simulink model "TST_AccPed_DrvDemLead"  (R2016b)
settings: Solver=FixedStepDiscrete  StartTime=0.0  StopTime=simTime  FixedStep=sampleTime  RelTol=1e-3
values from neighbouring files (symbols this model uses):
  testCase = 1    [initTST_AccPed_DrvDemLead_001.m]    (also in initTST_AccPed_DrvDemLead_002.m = 2; initTST_AccPed_DrvDemLead_003.m = 3; initTST_AccPed_DrvDemLead_004.m = 4)
libraries: simulink x17, UnitTest_Lib x12
settings Model: Creator=zhengjinyan  LastModifiedBy=zhengjinyan
settings DebuggingCC: SignalRangeChecking=error

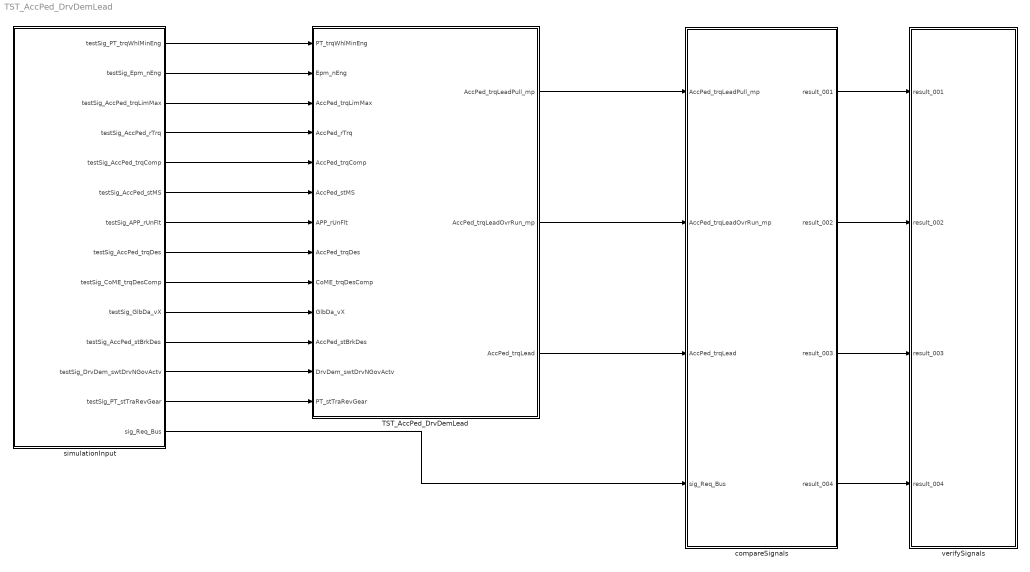
== system TST_AccPed_DrvDemLead ==
  TST_AccPed_DrvDemLead : Subsystem
  compareSignals : Subsystem
  simulationInput : Subsystem
  verifySignals : Subsystem
  wires:
  simulationInput/1(testSig_PT_trqWhlMinEng) -> TST_AccPed_DrvDemLead/1(PT_trqWhlMinEng)
  simulationInput/2(testSig_Epm_nEng) -> TST_AccPed_DrvDemLead/2(Epm_nEng)
  simulationInput/3(testSig_AccPed_trqLimMax) -> TST_AccPed_DrvDemLead/3(AccPed_trqLimMax)
  simulationInput/4(testSig_AccPed_rTrq) -> TST_AccPed_DrvDemLead/4(AccPed_rTrq)
  simulationInput/5(testSig_AccPed_trqComp) -> TST_AccPed_DrvDemLead/5(AccPed_trqComp)
  simulationInput/6(testSig_AccPed_stMS) -> TST_AccPed_DrvDemLead/6(AccPed_stMS)
  simulationInput/7(testSig_APP_rUnFlt) -> TST_AccPed_DrvDemLead/7(APP_rUnFlt)
  simulationInput/8(testSig_AccPed_trqDes) -> TST_AccPed_DrvDemLead/8(AccPed_trqDes)
  simulationInput/9(testSig_CoME_trqDesComp) -> TST_AccPed_DrvDemLead/9(CoME_trqDesComp)
  simulationInput/10(testSig_GlbDa_vX) -> TST_AccPed_DrvDemLead/10(GlbDa_vX)
  simulationInput/11(testSig_AccPed_stBrkDes) -> TST_AccPed_DrvDemLead/11(AccPed_stBrkDes)
  simulationInput/12(testSig_DrvDem_swtDrvNGovActv) -> TST_AccPed_DrvDemLead/12(DrvDem_swtDrvNGovActv)
  simulationInput/13(testSig_PT_stTraRevGear) -> TST_AccPed_DrvDemLead/13(PT_stTraRevGear)
  TST_AccPed_DrvDemLead/1(AccPed_trqLeadPull_mp) -> compareSignals/1(AccPed_trqLeadPull_mp)
  TST_AccPed_DrvDemLead/2(AccPed_trqLeadOvrRun_mp) -> compareSignals/2(AccPed_trqLeadOvrRun_mp)
  TST_AccPed_DrvDemLead/3(AccPed_trqLead) -> compareSignals/3(AccPed_trqLead)
  simulationInput/14(sig_Req_Bus) -> compareSignals/4(sig_Req_Bus)
  compareSignals/1(result_001) -> verifySignals/1(result_001)
  compareSignals/2(result_002) -> verifySignals/2(result_002)
  compareSignals/3(result_003) -> verifySignals/3(result_003)
  compareSignals/4(result_004) -> verifySignals/4(result_004)

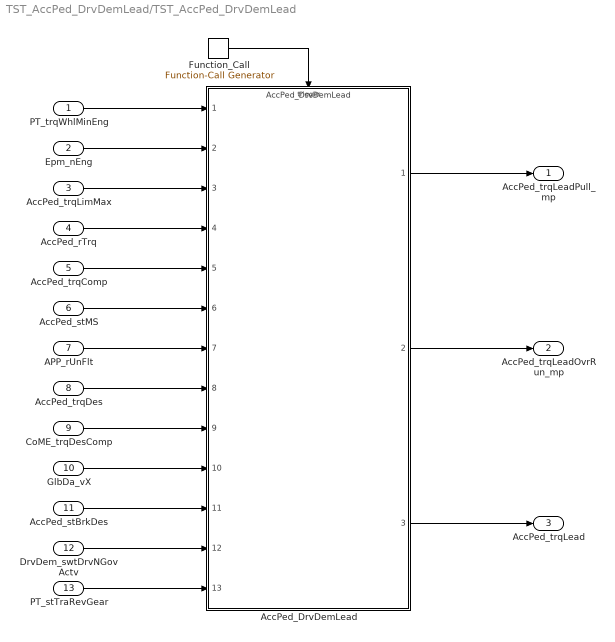
== system TST_AccPed_DrvDemLead/TST_AccPed_DrvDemLead ==
  PT_trqWhlMinEng : Inport
  Epm_nEng : Inport  Port=2
  AccPed_trqLimMax : Inport  Port=3
  AccPed_rTrq : Inport  Port=4
  AccPed_trqComp : Inport  Port=5
  AccPed_stMS : Inport  Port=6
  APP_rUnFlt : Inport  Port=7
  AccPed_trqDes : Inport  Port=8
  CoME_trqDesComp : Inport  Port=9
  GlbDa_vX : Inport  Port=10
  AccPed_stBrkDes : Inport  Port=11
  DrvDem_swtDrvNGovActv : Inport  Port=12
  PT_stTraRevGear : Inport  Port=13
  AccPed_DrvDemLead : ModelReference  ModelNameDialog=AccPed_DrvDemLead  SimulationMode=Normal  ModelReferenceVersion=1.27  TriggerPortName=function  TriggerPortTriggerType=function-call  TriggerPortStatesWhenEnabling=held
  Function_Call : simulink/Ports & Subsystems/Function-Call Generator  sample_time=sampleTime  numberOfIterations=1
  AccPed_trqLeadPull_mp : Outport
  AccPed_trqLeadOvrRun_mp : Outport  Port=2
  AccPed_trqLead : Outport  Port=3
  wires:
  Function_Call/1 -> AccPed_DrvDemLead/Trigger
  PT_trqWhlMinEng/1 -> AccPed_DrvDemLead/1
  Epm_nEng/1 -> AccPed_DrvDemLead/2
  AccPed_trqLimMax/1 -> AccPed_DrvDemLead/3
  AccPed_rTrq/1 -> AccPed_DrvDemLead/4
  AccPed_trqComp/1 -> AccPed_DrvDemLead/5
  AccPed_stMS/1 -> AccPed_DrvDemLead/6
  APP_rUnFlt/1 -> AccPed_DrvDemLead/7
  AccPed_trqDes/1 -> AccPed_DrvDemLead/8
  CoME_trqDesComp/1 -> AccPed_DrvDemLead/9
  GlbDa_vX/1 -> AccPed_DrvDemLead/10
  AccPed_stBrkDes/1 -> AccPed_DrvDemLead/11
  DrvDem_swtDrvNGovActv/1 -> AccPed_DrvDemLead/12
  PT_stTraRevGear/1 -> AccPed_DrvDemLead/13
  AccPed_DrvDemLead/1 -> AccPed_trqLeadPull_mp/1
  AccPed_DrvDemLead/2 -> AccPed_trqLeadOvrRun_mp/1
  AccPed_DrvDemLead/3 -> AccPed_trqLead/1

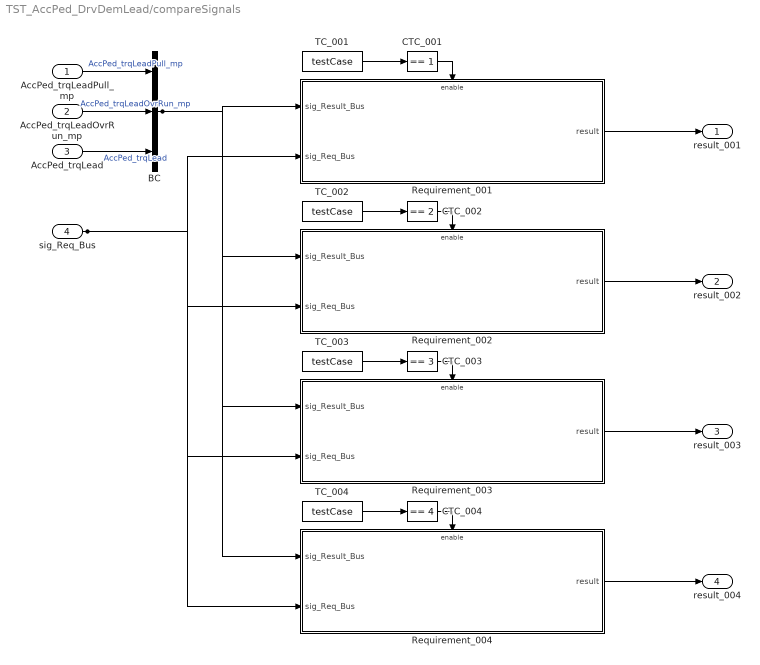
== system TST_AccPed_DrvDemLead/compareSignals ==
  AccPed_trqLeadPull_mp : Inport
  AccPed_trqLeadOvrRun_mp : Inport  Port=2
  AccPed_trqLead : Inport  Port=3
  sig_Req_Bus : Inport  Port=4
  BC : BusCreator  Inputs=3
  CTC_001 : simulink/Logic and Bit Operations/Compare To Constant  relop===  const=1  OutDataTypeStr=boolean
  CTC_002 : simulink/Logic and Bit Operations/Compare To Constant  relop===  const=2  OutDataTypeStr=boolean
  CTC_003 : simulink/Logic and Bit Operations/Compare To Constant  relop===  const=3  OutDataTypeStr=boolean
  CTC_004 : simulink/Logic and Bit Operations/Compare To Constant  relop===  const=4  OutDataTypeStr=boolean
  Requirement_001 : Subsystem
  Requirement_002 : Subsystem
  Requirement_003 : Subsystem
  Requirement_004 : Subsystem
  TC_001 : Constant  Value=testCase
  TC_002 : Constant  Value=testCase
  TC_003 : Constant  Value=testCase
  TC_004 : Constant  Value=testCase
  result_001 : Outport
  result_002 : Outport  Port=2
  result_003 : Outport  Port=3
  result_004 : Outport  Port=4
  wires:
  AccPed_trqLeadPull_mp/1 -> BC/1  "AccPed_trqLeadPull_mp"
  AccPed_trqLeadOvrRun_mp/1 -> BC/2  "AccPed_trqLeadOvrRun_mp"
  AccPed_trqLead/1 -> BC/3  "AccPed_trqLead"
  TC_001/1 -> CTC_001/1
  CTC_001/1 -> Requirement_001/Enable
  sig_Req_Bus/1 -> Requirement_001/2(sig_Req_Bus), Requirement_002/2(sig_Req_Bus), Requirement_003/2(sig_Req_Bus), Requirement_004/2(sig_Req_Bus)
  BC/1 -> Requirement_001/1(sig_Result_Bus), Requirement_002/1(sig_Result_Bus), Requirement_003/1(sig_Result_Bus), Requirement_004/1(sig_Result_Bus)
  Requirement_001/1(result) -> result_001/1
  TC_002/1 -> CTC_002/1
  CTC_002/1 -> Requirement_002/Enable
  Requirement_002/1(result) -> result_002/1
  TC_003/1 -> CTC_003/1
  CTC_003/1 -> Requirement_003/Enable
  Requirement_003/1(result) -> result_003/1
  TC_004/1 -> CTC_004/1
  CTC_004/1 -> Requirement_004/Enable
  Requirement_004/1(result) -> result_004/1

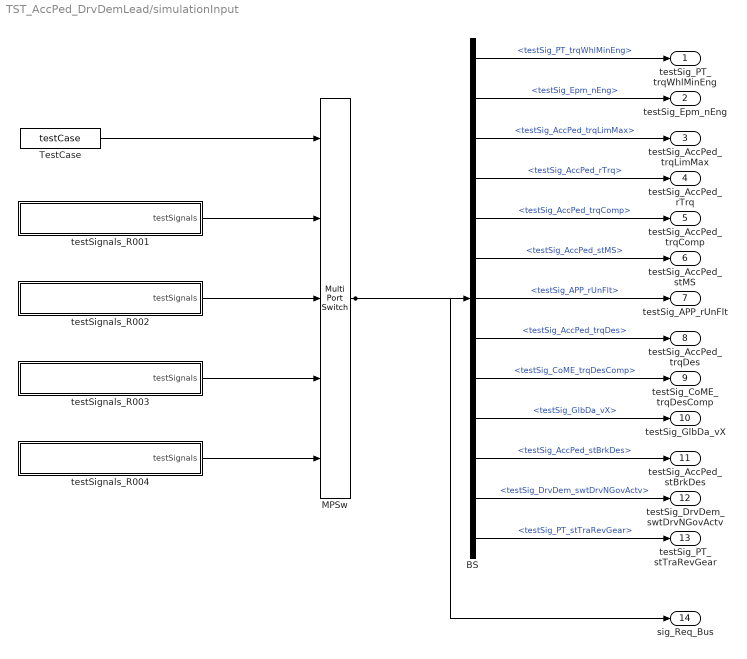
== system TST_AccPed_DrvDemLead/simulationInput ==
  BS : BusSelector  OutputSignals=testSig_PT_trqWhlMinEng,testSig_Epm_nEng,testSig_AccPed_trqLimMax,testSig_AccPed_rTrq,testSig_AccPed_trqComp,testSig_AccPed_stMS,testSig_APP_rUnFlt,testSig_AccPed_trqDes,testSig_CoME_trqDesComp,testSig_GlbDa_vX,testSig_AccPed_stBrkDes,testSig_DrvDem_swtDrvNGovActv,testSig_PT_stTraRevGear
  MPSw : MultiPortSwitch  Inputs=4  SaturateOnIntegerOverflow=on  InputSameDT=on
  TestCase : Constant  Value=testCase
  testSignals_R001 : Subsystem
  testSignals_R002 : Subsystem
  testSignals_R003 : Subsystem
  testSignals_R004 : Subsystem
  testSig_PT_trqWhlMinEng : Outport
  testSig_Epm_nEng : Outport  Port=2
  testSig_AccPed_trqLimMax : Outport  Port=3
  testSig_AccPed_rTrq : Outport  Port=4
  testSig_AccPed_trqComp : Outport  Port=5
  testSig_AccPed_stMS : Outport  Port=6
  testSig_APP_rUnFlt : Outport  Port=7
  testSig_AccPed_trqDes : Outport  Port=8
  testSig_CoME_trqDesComp : Outport  Port=9
  testSig_GlbDa_vX : Outport  Port=10
  testSig_AccPed_stBrkDes : Outport  Port=11
  testSig_DrvDem_swtDrvNGovActv : Outport  Port=12
  testSig_PT_stTraRevGear : Outport  Port=13
  sig_Req_Bus : Outport  Port=14
  wires:
  BS/1 -> testSig_PT_trqWhlMinEng/1  "<testSig_PT_trqWhlMinEng>"
  BS/2 -> testSig_Epm_nEng/1  "<testSig_Epm_nEng>"
  BS/3 -> testSig_AccPed_trqLimMax/1  "<testSig_AccPed_trqLimMax>"
  BS/4 -> testSig_AccPed_rTrq/1  "<testSig_AccPed_rTrq>"
  BS/5 -> testSig_AccPed_trqComp/1  "<testSig_AccPed_trqComp>"
  BS/6 -> testSig_AccPed_stMS/1  "<testSig_AccPed_stMS>"
  BS/7 -> testSig_APP_rUnFlt/1  "<testSig_APP_rUnFlt>"
  BS/8 -> testSig_AccPed_trqDes/1  "<testSig_AccPed_trqDes>"
  BS/9 -> testSig_CoME_trqDesComp/1  "<testSig_CoME_trqDesComp>"
  BS/10 -> testSig_GlbDa_vX/1  "<testSig_GlbDa_vX>"
  BS/11 -> testSig_AccPed_stBrkDes/1  "<testSig_AccPed_stBrkDes>"
  BS/12 -> testSig_DrvDem_swtDrvNGovActv/1  "<testSig_DrvDem_swtDrvNGovActv>"
  BS/13 -> testSig_PT_stTraRevGear/1  "<testSig_PT_stTraRevGear>"
  MPSw/1 -> BS/1, sig_Req_Bus/1
  TestCase/1 -> MPSw/1
  testSignals_R001/1(testSignals) -> MPSw/2
  testSignals_R002/1(testSignals) -> MPSw/3
  testSignals_R003/1(testSignals) -> MPSw/4
  testSignals_R004/1(testSignals) -> MPSw/5

== system TST_AccPed_DrvDemLead/verifySignals ==
  result_001 : Inport
  result_002 : Inport  Port=2
  result_003 : Inport  Port=3
  result_004 : Inport  Port=4
  Assertion_001 : Assertion  Enabled=off
  Assertion_002 : Assertion  Enabled=off
  Assertion_003 : Assertion  Enabled=off
  Assertion_004 : Assertion  Enabled=off
  wires:
  result_001/1 -> Assertion_001/1
  result_002/1 -> Assertion_002/1
  result_003/1 -> Assertion_003/1
  result_004/1 -> Assertion_004/1

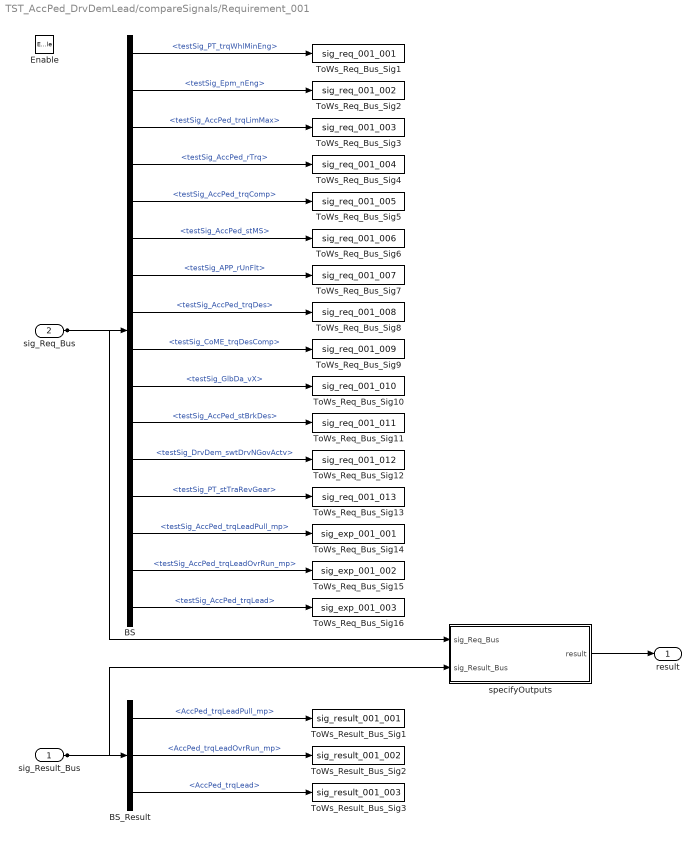
== system TST_AccPed_DrvDemLead/compareSignals/Requirement_001 ==
  sig_Result_Bus : Inport
  sig_Req_Bus : Inport  Port=2
  Enable : EnablePort
  BS : BusSelector  OutputSignals=testSig_PT_trqWhlMinEng,testSig_Epm_nEng,testSig_AccPed_trqLimMax,testSig_AccPed_rTrq,testSig_AccPed_trqComp,testSig_AccPed_stMS,testSig_APP_rUnFlt,testSig_AccPed_trqDes,testSig_CoME_trqDesComp,testSig_GlbDa_vX,testSig_AccPed_stBrkDes,testSig_DrvDem_swtDrvNGovActv,testSig_PT_stTraRevGear,testSig_AccPed_trqLeadPull_mp,testSig_AccPed_trqLeadOvrRun_mp,testSig_AccPed_trqLead
  BS_Result : BusSelector  OutputSignals=AccPed_trqLeadPull_mp,AccPed_trqLeadOvrRun_mp,AccPed_trqLead
  ToWs_Req_Bus_Sig1 : ToWorkspace  VariableName=sig_req_001_001  SaveFormat=Structure With Time
  ToWs_Req_Bus_Sig10 : ToWorkspace  VariableName=sig_req_001_010  SaveFormat=Structure With Time
  ToWs_Req_Bus_Sig11 : ToWorkspace  VariableName=sig_req_001_011  SaveFormat=Structure With Time
  ToWs_Req_Bus_Sig12 : ToWorkspace  VariableName=sig_req_001_012  SaveFormat=Structure With Time
  ToWs_Req_Bus_Sig13 : ToWorkspace  VariableName=sig_req_001_013  SaveFormat=Structure With Time
  ToWs_Req_Bus_Sig14 : ToWorkspace  VariableName=sig_exp_001_001  SaveFormat=Structure With Time
  ToWs_Req_Bus_Sig15 : ToWorkspace  VariableName=sig_exp_001_002  SaveFormat=Structure With Time
  ToWs_Req_Bus_Sig16 : ToWorkspace  VariableName=sig_exp_001_003  SaveFormat=Structure With Time
  ToWs_Req_Bus_Sig2 : ToWorkspace  VariableName=sig_req_001_002  SaveFormat=Structure With Time
  ToWs_Req_Bus_Sig3 : ToWorkspace  VariableName=sig_req_001_003  SaveFormat=Structure With Time
  ToWs_Req_Bus_Sig4 : ToWorkspace  VariableName=sig_req_001_004  SaveFormat=Structure With Time
  ToWs_Req_Bus_Sig5 : ToWorkspace  VariableName=sig_req_001_005  SaveFormat=Structure With Time
  ToWs_Req_Bus_Sig6 : ToWorkspace  VariableName=sig_req_001_006  SaveFormat=Structure With Time
  ToWs_Req_Bus_Sig7 : ToWorkspace  VariableName=sig_req_001_007  SaveFormat=Structure With Time
  ToWs_Req_Bus_Sig8 : ToWorkspace  VariableName=sig_req_001_008  SaveFormat=Structure With Time
  ToWs_Req_Bus_Sig9 : ToWorkspace  VariableName=sig_req_001_009  SaveFormat=Structure With Time
  ToWs_Result_Bus_Sig1 : ToWorkspace  VariableName=sig_result_001_001  SaveFormat=Structure With Time
  ToWs_Result_Bus_Sig2 : ToWorkspace  VariableName=sig_result_001_002  SaveFormat=Structure With Time
  ToWs_Result_Bus_Sig3 : ToWorkspace  VariableName=sig_result_001_003  SaveFormat=Structure With Time
  specifyOutputs : Subsystem
  result : Outport
  wires:
  sig_Req_Bus/1 -> BS/1, specifyOutputs/1(sig_Req_Bus)
  BS/1 -> ToWs_Req_Bus_Sig1/1  "<testSig_PT_trqWhlMinEng>"
  BS/2 -> ToWs_Req_Bus_Sig2/1  "<testSig_Epm_nEng>"
  BS/3 -> ToWs_Req_Bus_Sig3/1  "<testSig_AccPed_trqLimMax>"
  BS/4 -> ToWs_Req_Bus_Sig4/1  "<testSig_AccPed_rTrq>"
  BS/5 -> ToWs_Req_Bus_Sig5/1  "<testSig_AccPed_trqComp>"
  BS/6 -> ToWs_Req_Bus_Sig6/1  "<testSig_AccPed_stMS>"
  BS/7 -> ToWs_Req_Bus_Sig7/1  "<testSig_APP_rUnFlt>"
  BS/8 -> ToWs_Req_Bus_Sig8/1  "<testSig_AccPed_trqDes>"
  BS/9 -> ToWs_Req_Bus_Sig9/1  "<testSig_CoME_trqDesComp>"
  BS/10 -> ToWs_Req_Bus_Sig10/1  "<testSig_GlbDa_vX>"
  BS/11 -> ToWs_Req_Bus_Sig11/1  "<testSig_AccPed_stBrkDes>"
  BS/12 -> ToWs_Req_Bus_Sig12/1  "<testSig_DrvDem_swtDrvNGovActv>"
  BS/13 -> ToWs_Req_Bus_Sig13/1  "<testSig_PT_stTraRevGear>"
  BS/14 -> ToWs_Req_Bus_Sig14/1  "<testSig_AccPed_trqLeadPull_mp>"
  BS/15 -> ToWs_Req_Bus_Sig15/1  "<testSig_AccPed_trqLeadOvrRun_mp>"
  BS/16 -> ToWs_Req_Bus_Sig16/1  "<testSig_AccPed_trqLead>"
  sig_Result_Bus/1 -> BS_Result/1, specifyOutputs/2(sig_Result_Bus)
  BS_Result/1 -> ToWs_Result_Bus_Sig1/1  "<AccPed_trqLeadPull_mp>"
  BS_Result/2 -> ToWs_Result_Bus_Sig2/1  "<AccPed_trqLeadOvrRun_mp>"
  BS_Result/3 -> ToWs_Result_Bus_Sig3/1  "<AccPed_trqLead>"
  specifyOutputs/1(result) -> result/1

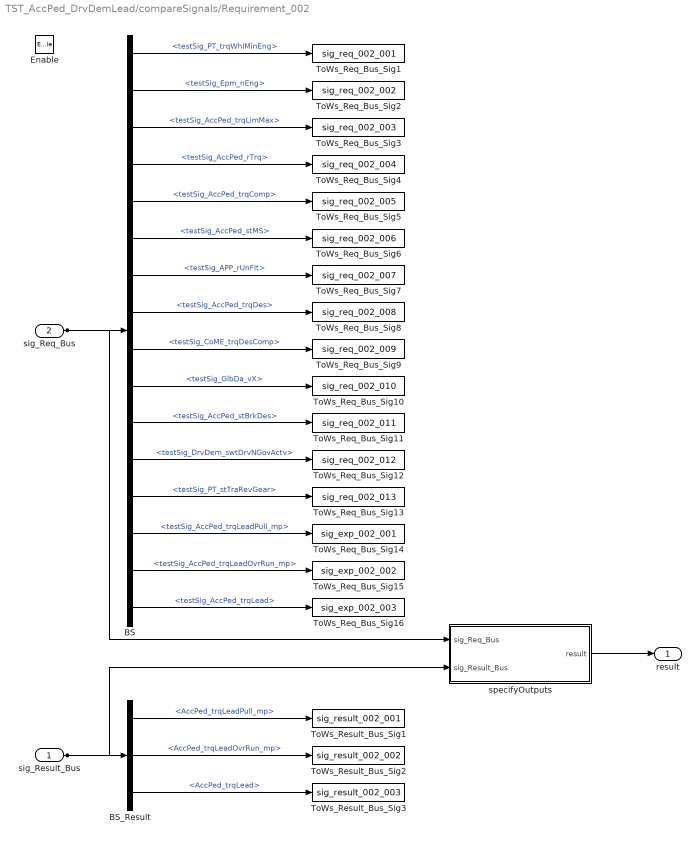
== system TST_AccPed_DrvDemLead/compareSignals/Requirement_002 ==
  sig_Result_Bus : Inport
  sig_Req_Bus : Inport  Port=2
  Enable : EnablePort
  BS : BusSelector  OutputSignals=testSig_PT_trqWhlMinEng,testSig_Epm_nEng,testSig_AccPed_trqLimMax,testSig_AccPed_rTrq,testSig_AccPed_trqComp,testSig_AccPed_stMS,testSig_APP_rUnFlt,testSig_AccPed_trqDes,testSig_CoME_trqDesComp,testSig_GlbDa_vX,testSig_AccPed_stBrkDes,testSig_DrvDem_swtDrvNGovActv,testSig_PT_stTraRevGear,testSig_AccPed_trqLeadPull_mp,testSig_AccPed_trqLeadOvrRun_mp,testSig_AccPed_trqLead
  BS_Result : BusSelector  OutputSignals=AccPed_trqLeadPull_mp,AccPed_trqLeadOvrRun_mp,AccPed_trqLead
  ToWs_Req_Bus_Sig1 : ToWorkspace  VariableName=sig_req_002_001  SaveFormat=Structure With Time
  ToWs_Req_Bus_Sig10 : ToWorkspace  VariableName=sig_req_002_010  SaveFormat=Structure With Time
  ToWs_Req_Bus_Sig11 : ToWorkspace  VariableName=sig_req_002_011  SaveFormat=Structure With Time
  ToWs_Req_Bus_Sig12 : ToWorkspace  VariableName=sig_req_002_012  SaveFormat=Structure With Time
  ToWs_Req_Bus_Sig13 : ToWorkspace  VariableName=sig_req_002_013  SaveFormat=Structure With Time
  ToWs_Req_Bus_Sig14 : ToWorkspace  VariableName=sig_exp_002_001  SaveFormat=Structure With Time
  ToWs_Req_Bus_Sig15 : ToWorkspace  VariableName=sig_exp_002_002  SaveFormat=Structure With Time
  ToWs_Req_Bus_Sig16 : ToWorkspace  VariableName=sig_exp_002_003  SaveFormat=Structure With Time
  ToWs_Req_Bus_Sig2 : ToWorkspace  VariableName=sig_req_002_002  SaveFormat=Structure With Time
  ToWs_Req_Bus_Sig3 : ToWorkspace  VariableName=sig_req_002_003  SaveFormat=Structure With Time
  ToWs_Req_Bus_Sig4 : ToWorkspace  VariableName=sig_req_002_004  SaveFormat=Structure With Time
  ToWs_Req_Bus_Sig5 : ToWorkspace  VariableName=sig_req_002_005  SaveFormat=Structure With Time
  ToWs_Req_Bus_Sig6 : ToWorkspace  VariableName=sig_req_002_006  SaveFormat=Structure With Time
  ToWs_Req_Bus_Sig7 : ToWorkspace  VariableName=sig_req_002_007  SaveFormat=Structure With Time
  ToWs_Req_Bus_Sig8 : ToWorkspace  VariableName=sig_req_002_008  SaveFormat=Structure With Time
  ToWs_Req_Bus_Sig9 : ToWorkspace  VariableName=sig_req_002_009  SaveFormat=Structure With Time
  ToWs_Result_Bus_Sig1 : ToWorkspace  VariableName=sig_result_002_001  SaveFormat=Structure With Time
  ToWs_Result_Bus_Sig2 : ToWorkspace  VariableName=sig_result_002_002  SaveFormat=Structure With Time
  ToWs_Result_Bus_Sig3 : ToWorkspace  VariableName=sig_result_002_003  SaveFormat=Structure With Time
  specifyOutputs : Subsystem
  result : Outport
  wires:
  sig_Req_Bus/1 -> BS/1, specifyOutputs/1(sig_Req_Bus)
  BS/1 -> ToWs_Req_Bus_Sig1/1  "<testSig_PT_trqWhlMinEng>"
  BS/2 -> ToWs_Req_Bus_Sig2/1  "<testSig_Epm_nEng>"
  BS/3 -> ToWs_Req_Bus_Sig3/1  "<testSig_AccPed_trqLimMax>"
  BS/4 -> ToWs_Req_Bus_Sig4/1  "<testSig_AccPed_rTrq>"
  BS/5 -> ToWs_Req_Bus_Sig5/1  "<testSig_AccPed_trqComp>"
  BS/6 -> ToWs_Req_Bus_Sig6/1  "<testSig_AccPed_stMS>"
  BS/7 -> ToWs_Req_Bus_Sig7/1  "<testSig_APP_rUnFlt>"
  BS/8 -> ToWs_Req_Bus_Sig8/1  "<testSig_AccPed_trqDes>"
  BS/9 -> ToWs_Req_Bus_Sig9/1  "<testSig_CoME_trqDesComp>"
  BS/10 -> ToWs_Req_Bus_Sig10/1  "<testSig_GlbDa_vX>"
  BS/11 -> ToWs_Req_Bus_Sig11/1  "<testSig_AccPed_stBrkDes>"
  BS/12 -> ToWs_Req_Bus_Sig12/1  "<testSig_DrvDem_swtDrvNGovActv>"
  BS/13 -> ToWs_Req_Bus_Sig13/1  "<testSig_PT_stTraRevGear>"
  BS/14 -> ToWs_Req_Bus_Sig14/1  "<testSig_AccPed_trqLeadPull_mp>"
  BS/15 -> ToWs_Req_Bus_Sig15/1  "<testSig_AccPed_trqLeadOvrRun_mp>"
  BS/16 -> ToWs_Req_Bus_Sig16/1  "<testSig_AccPed_trqLead>"
  sig_Result_Bus/1 -> BS_Result/1, specifyOutputs/2(sig_Result_Bus)
  BS_Result/1 -> ToWs_Result_Bus_Sig1/1  "<AccPed_trqLeadPull_mp>"
  BS_Result/2 -> ToWs_Result_Bus_Sig2/1  "<AccPed_trqLeadOvrRun_mp>"
  BS_Result/3 -> ToWs_Result_Bus_Sig3/1  "<AccPed_trqLead>"
  specifyOutputs/1(result) -> result/1

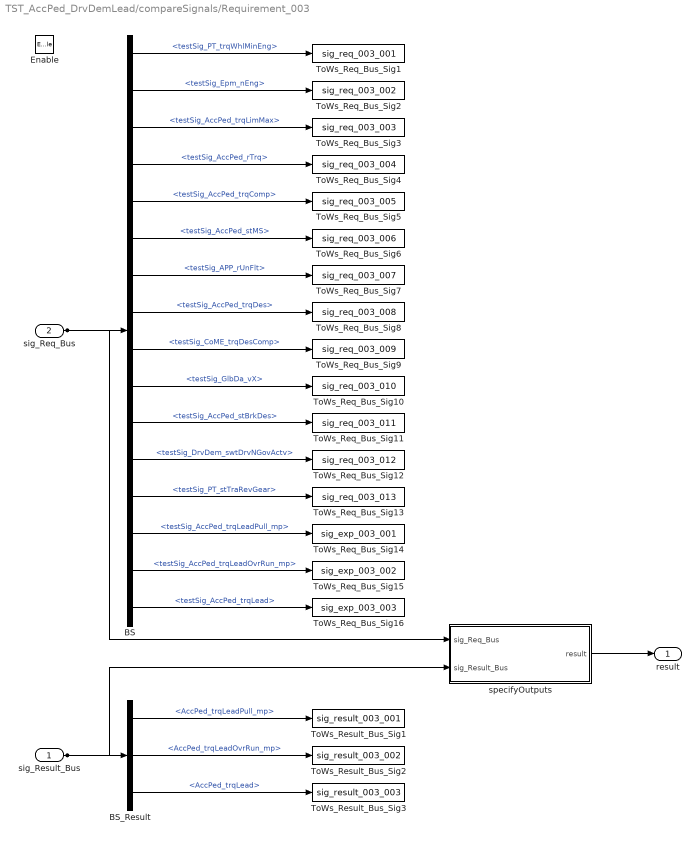
== system TST_AccPed_DrvDemLead/compareSignals/Requirement_003 ==
  sig_Result_Bus : Inport
  sig_Req_Bus : Inport  Port=2
  Enable : EnablePort
  BS : BusSelector  OutputSignals=testSig_PT_trqWhlMinEng,testSig_Epm_nEng,testSig_AccPed_trqLimMax,testSig_AccPed_rTrq,testSig_AccPed_trqComp,testSig_AccPed_stMS,testSig_APP_rUnFlt,testSig_AccPed_trqDes,testSig_CoME_trqDesComp,testSig_GlbDa_vX,testSig_AccPed_stBrkDes,testSig_DrvDem_swtDrvNGovActv,testSig_PT_stTraRevGear,testSig_AccPed_trqLeadPull_mp,testSig_AccPed_trqLeadOvrRun_mp,testSig_AccPed_trqLead
  BS_Result : BusSelector  OutputSignals=AccPed_trqLeadPull_mp,AccPed_trqLeadOvrRun_mp,AccPed_trqLead
  ToWs_Req_Bus_Sig1 : ToWorkspace  VariableName=sig_req_003_001  SaveFormat=Structure With Time
  ToWs_Req_Bus_Sig10 : ToWorkspace  VariableName=sig_req_003_010  SaveFormat=Structure With Time
  ToWs_Req_Bus_Sig11 : ToWorkspace  VariableName=sig_req_003_011  SaveFormat=Structure With Time
  ToWs_Req_Bus_Sig12 : ToWorkspace  VariableName=sig_req_003_012  SaveFormat=Structure With Time
  ToWs_Req_Bus_Sig13 : ToWorkspace  VariableName=sig_req_003_013  SaveFormat=Structure With Time
  ToWs_Req_Bus_Sig14 : ToWorkspace  VariableName=sig_exp_003_001  SaveFormat=Structure With Time
  ToWs_Req_Bus_Sig15 : ToWorkspace  VariableName=sig_exp_003_002  SaveFormat=Structure With Time
  ToWs_Req_Bus_Sig16 : ToWorkspace  VariableName=sig_exp_003_003  SaveFormat=Structure With Time
  ToWs_Req_Bus_Sig2 : ToWorkspace  VariableName=sig_req_003_002  SaveFormat=Structure With Time
  ToWs_Req_Bus_Sig3 : ToWorkspace  VariableName=sig_req_003_003  SaveFormat=Structure With Time
  ToWs_Req_Bus_Sig4 : ToWorkspace  VariableName=sig_req_003_004  SaveFormat=Structure With Time
  ToWs_Req_Bus_Sig5 : ToWorkspace  VariableName=sig_req_003_005  SaveFormat=Structure With Time
  ToWs_Req_Bus_Sig6 : ToWorkspace  VariableName=sig_req_003_006  SaveFormat=Structure With Time
  ToWs_Req_Bus_Sig7 : ToWorkspace  VariableName=sig_req_003_007  SaveFormat=Structure With Time
  ToWs_Req_Bus_Sig8 : ToWorkspace  VariableName=sig_req_003_008  SaveFormat=Structure With Time
  ToWs_Req_Bus_Sig9 : ToWorkspace  VariableName=sig_req_003_009  SaveFormat=Structure With Time
  ToWs_Result_Bus_Sig1 : ToWorkspace  VariableName=sig_result_003_001  SaveFormat=Structure With Time
  ToWs_Result_Bus_Sig2 : ToWorkspace  VariableName=sig_result_003_002  SaveFormat=Structure With Time
  ToWs_Result_Bus_Sig3 : ToWorkspace  VariableName=sig_result_003_003  SaveFormat=Structure With Time
  specifyOutputs : Subsystem
  result : Outport
  wires:
  sig_Req_Bus/1 -> BS/1, specifyOutputs/1(sig_Req_Bus)
  BS/1 -> ToWs_Req_Bus_Sig1/1  "<testSig_PT_trqWhlMinEng>"
  BS/2 -> ToWs_Req_Bus_Sig2/1  "<testSig_Epm_nEng>"
  BS/3 -> ToWs_Req_Bus_Sig3/1  "<testSig_AccPed_trqLimMax>"
  BS/4 -> ToWs_Req_Bus_Sig4/1  "<testSig_AccPed_rTrq>"
  BS/5 -> ToWs_Req_Bus_Sig5/1  "<testSig_AccPed_trqComp>"
  BS/6 -> ToWs_Req_Bus_Sig6/1  "<testSig_AccPed_stMS>"
  BS/7 -> ToWs_Req_Bus_Sig7/1  "<testSig_APP_rUnFlt>"
  BS/8 -> ToWs_Req_Bus_Sig8/1  "<testSig_AccPed_trqDes>"
  BS/9 -> ToWs_Req_Bus_Sig9/1  "<testSig_CoME_trqDesComp>"
  BS/10 -> ToWs_Req_Bus_Sig10/1  "<testSig_GlbDa_vX>"
  BS/11 -> ToWs_Req_Bus_Sig11/1  "<testSig_AccPed_stBrkDes>"
  BS/12 -> ToWs_Req_Bus_Sig12/1  "<testSig_DrvDem_swtDrvNGovActv>"
  BS/13 -> ToWs_Req_Bus_Sig13/1  "<testSig_PT_stTraRevGear>"
  BS/14 -> ToWs_Req_Bus_Sig14/1  "<testSig_AccPed_trqLeadPull_mp>"
  BS/15 -> ToWs_Req_Bus_Sig15/1  "<testSig_AccPed_trqLeadOvrRun_mp>"
  BS/16 -> ToWs_Req_Bus_Sig16/1  "<testSig_AccPed_trqLead>"
  sig_Result_Bus/1 -> BS_Result/1, specifyOutputs/2(sig_Result_Bus)
  BS_Result/1 -> ToWs_Result_Bus_Sig1/1  "<AccPed_trqLeadPull_mp>"
  BS_Result/2 -> ToWs_Result_Bus_Sig2/1  "<AccPed_trqLeadOvrRun_mp>"
  BS_Result/3 -> ToWs_Result_Bus_Sig3/1  "<AccPed_trqLead>"
  specifyOutputs/1(result) -> result/1

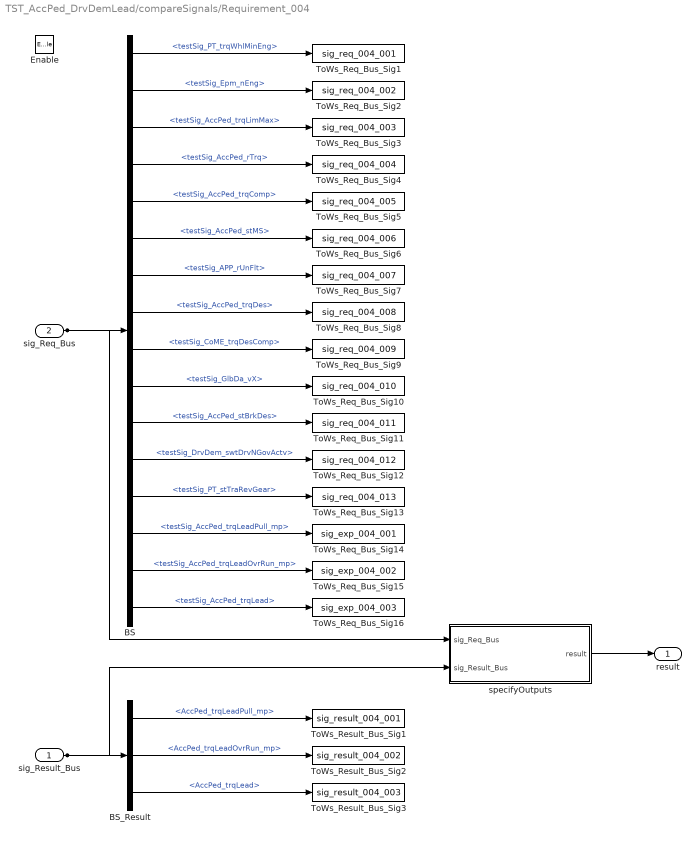
== system TST_AccPed_DrvDemLead/compareSignals/Requirement_004 ==
  sig_Result_Bus : Inport
  sig_Req_Bus : Inport  Port=2
  Enable : EnablePort
  BS : BusSelector  OutputSignals=testSig_PT_trqWhlMinEng,testSig_Epm_nEng,testSig_AccPed_trqLimMax,testSig_AccPed_rTrq,testSig_AccPed_trqComp,testSig_AccPed_stMS,testSig_APP_rUnFlt,testSig_AccPed_trqDes,testSig_CoME_trqDesComp,testSig_GlbDa_vX,testSig_AccPed_stBrkDes,testSig_DrvDem_swtDrvNGovActv,testSig_PT_stTraRevGear,testSig_AccPed_trqLeadPull_mp,testSig_AccPed_trqLeadOvrRun_mp,testSig_AccPed_trqLead
  BS_Result : BusSelector  OutputSignals=AccPed_trqLeadPull_mp,AccPed_trqLeadOvrRun_mp,AccPed_trqLead
  ToWs_Req_Bus_Sig1 : ToWorkspace  VariableName=sig_req_004_001  SaveFormat=Structure With Time
  ToWs_Req_Bus_Sig10 : ToWorkspace  VariableName=sig_req_004_010  SaveFormat=Structure With Time
  ToWs_Req_Bus_Sig11 : ToWorkspace  VariableName=sig_req_004_011  SaveFormat=Structure With Time
  ToWs_Req_Bus_Sig12 : ToWorkspace  VariableName=sig_req_004_012  SaveFormat=Structure With Time
  ToWs_Req_Bus_Sig13 : ToWorkspace  VariableName=sig_req_004_013  SaveFormat=Structure With Time
  ToWs_Req_Bus_Sig14 : ToWorkspace  VariableName=sig_exp_004_001  SaveFormat=Structure With Time
  ToWs_Req_Bus_Sig15 : ToWorkspace  VariableName=sig_exp_004_002  SaveFormat=Structure With Time
  ToWs_Req_Bus_Sig16 : ToWorkspace  VariableName=sig_exp_004_003  SaveFormat=Structure With Time
  ToWs_Req_Bus_Sig2 : ToWorkspace  VariableName=sig_req_004_002  SaveFormat=Structure With Time
  ToWs_Req_Bus_Sig3 : ToWorkspace  VariableName=sig_req_004_003  SaveFormat=Structure With Time
  ToWs_Req_Bus_Sig4 : ToWorkspace  VariableName=sig_req_004_004  SaveFormat=Structure With Time
  ToWs_Req_Bus_Sig5 : ToWorkspace  VariableName=sig_req_004_005  SaveFormat=Structure With Time
  ToWs_Req_Bus_Sig6 : ToWorkspace  VariableName=sig_req_004_006  SaveFormat=Structure With Time
  ToWs_Req_Bus_Sig7 : ToWorkspace  VariableName=sig_req_004_007  SaveFormat=Structure With Time
  ToWs_Req_Bus_Sig8 : ToWorkspace  VariableName=sig_req_004_008  SaveFormat=Structure With Time
  ToWs_Req_Bus_Sig9 : ToWorkspace  VariableName=sig_req_004_009  SaveFormat=Structure With Time
  ToWs_Result_Bus_Sig1 : ToWorkspace  VariableName=sig_result_004_001  SaveFormat=Structure With Time
  ToWs_Result_Bus_Sig2 : ToWorkspace  VariableName=sig_result_004_002  SaveFormat=Structure With Time
  ToWs_Result_Bus_Sig3 : ToWorkspace  VariableName=sig_result_004_003  SaveFormat=Structure With Time
  specifyOutputs : Subsystem
  result : Outport
  wires:
  sig_Req_Bus/1 -> BS/1, specifyOutputs/1(sig_Req_Bus)
  BS/1 -> ToWs_Req_Bus_Sig1/1  "<testSig_PT_trqWhlMinEng>"
  BS/2 -> ToWs_Req_Bus_Sig2/1  "<testSig_Epm_nEng>"
  BS/3 -> ToWs_Req_Bus_Sig3/1  "<testSig_AccPed_trqLimMax>"
  BS/4 -> ToWs_Req_Bus_Sig4/1  "<testSig_AccPed_rTrq>"
  BS/5 -> ToWs_Req_Bus_Sig5/1  "<testSig_AccPed_trqComp>"
  BS/6 -> ToWs_Req_Bus_Sig6/1  "<testSig_AccPed_stMS>"
  BS/7 -> ToWs_Req_Bus_Sig7/1  "<testSig_APP_rUnFlt>"
  BS/8 -> ToWs_Req_Bus_Sig8/1  "<testSig_AccPed_trqDes>"
  BS/9 -> ToWs_Req_Bus_Sig9/1  "<testSig_CoME_trqDesComp>"
  BS/10 -> ToWs_Req_Bus_Sig10/1  "<testSig_GlbDa_vX>"
  BS/11 -> ToWs_Req_Bus_Sig11/1  "<testSig_AccPed_stBrkDes>"
  BS/12 -> ToWs_Req_Bus_Sig12/1  "<testSig_DrvDem_swtDrvNGovActv>"
  BS/13 -> ToWs_Req_Bus_Sig13/1  "<testSig_PT_stTraRevGear>"
  BS/14 -> ToWs_Req_Bus_Sig14/1  "<testSig_AccPed_trqLeadPull_mp>"
  BS/15 -> ToWs_Req_Bus_Sig15/1  "<testSig_AccPed_trqLeadOvrRun_mp>"
  BS/16 -> ToWs_Req_Bus_Sig16/1  "<testSig_AccPed_trqLead>"
  sig_Result_Bus/1 -> BS_Result/1, specifyOutputs/2(sig_Result_Bus)
  BS_Result/1 -> ToWs_Result_Bus_Sig1/1  "<AccPed_trqLeadPull_mp>"
  BS_Result/2 -> ToWs_Result_Bus_Sig2/1  "<AccPed_trqLeadOvrRun_mp>"
  BS_Result/3 -> ToWs_Result_Bus_Sig3/1  "<AccPed_trqLead>"
  specifyOutputs/1(result) -> result/1

== system TST_AccPed_DrvDemLead/simulationInput/testSignals_R001 ==
  BC : BusCreator  Inputs=16
  spec_APP_rUnFlt : FromWorkspace  VariableName=testSig_APP_rUnFlt  Interpolate=off  OutputAfterFinalValue=Holding final value
  spec_AccPed_rTrq : FromWorkspace  VariableName=testSig_AccPed_rTrq  Interpolate=off  OutputAfterFinalValue=Holding final value
  spec_AccPed_stBrkDes : FromWorkspace  VariableName=testSig_AccPed_stBrkDes  Interpolate=off  OutputAfterFinalValue=Holding final value
  spec_AccPed_stMS : FromWorkspace  VariableName=testSig_AccPed_stMS  Interpolate=off  OutputAfterFinalValue=Holding final value
  spec_AccPed_trqComp : FromWorkspace  VariableName=testSig_AccPed_trqComp  Interpolate=off  OutputAfterFinalValue=Holding final value
  spec_AccPed_trqDes : FromWorkspace  VariableName=testSig_AccPed_trqDes  Interpolate=off  OutputAfterFinalValue=Holding final value
  spec_AccPed_trqLead : FromWorkspace  VariableName=testSig_AccPed_trqLead  Interpolate=off  OutputAfterFinalValue=Holding final value
  spec_AccPed_trqLeadOvrRun_mp : FromWorkspace  VariableName=testSig_AccPed_trqLeadOvrRun_mp  Interpolate=off  OutputAfterFinalValue=Holding final value
  spec_AccPed_trqLeadPull_mp : FromWorkspace  VariableName=testSig_AccPed_trqLeadPull_mp  Interpolate=off  OutputAfterFinalValue=Holding final value
  spec_AccPed_trqLimMax : FromWorkspace  VariableName=testSig_AccPed_trqLimMax  Interpolate=off  OutputAfterFinalValue=Holding final value
  spec_CoME_trqDesComp : FromWorkspace  VariableName=testSig_CoME_trqDesComp  Interpolate=off  OutputAfterFinalValue=Holding final value
  spec_DrvDem_swtDrvNGovActv : FromWorkspace  VariableName=testSig_DrvDem_swtDrvNGovActv  Interpolate=off  OutputAfterFinalValue=Holding final value
  spec_Epm_nEng : FromWorkspace  VariableName=testSig_Epm_nEng  Interpolate=off  OutputAfterFinalValue=Holding final value
  spec_GlbDa_vX : FromWorkspace  VariableName=testSig_GlbDa_vX  Interpolate=off  OutputAfterFinalValue=Holding final value
  spec_PT_stTraRevGear : FromWorkspace  VariableName=testSig_PT_stTraRevGear  Interpolate=off  OutputAfterFinalValue=Holding final value
  spec_PT_trqWhlMinEng : FromWorkspace  VariableName=testSig_PT_trqWhlMinEng  Interpolate=off  OutputAfterFinalValue=Holding final value
  testSignals : Outport
  wires:
  BC/1 -> testSignals/1
  spec_PT_trqWhlMinEng/1 -> BC/1  "testSig_PT_trqWhlMinEng"
  spec_Epm_nEng/1 -> BC/2  "testSig_Epm_nEng"
  spec_AccPed_trqLimMax/1 -> BC/3  "testSig_AccPed_trqLimMax"
  spec_AccPed_rTrq/1 -> BC/4  "testSig_AccPed_rTrq"
  spec_AccPed_trqComp/1 -> BC/5  "testSig_AccPed_trqComp"
  spec_AccPed_stMS/1 -> BC/6  "testSig_AccPed_stMS"
  spec_APP_rUnFlt/1 -> BC/7  "testSig_APP_rUnFlt"
  spec_AccPed_trqDes/1 -> BC/8  "testSig_AccPed_trqDes"
  spec_CoME_trqDesComp/1 -> BC/9  "testSig_CoME_trqDesComp"
  spec_GlbDa_vX/1 -> BC/10  "testSig_GlbDa_vX"
  spec_AccPed_stBrkDes/1 -> BC/11  "testSig_AccPed_stBrkDes"
  spec_DrvDem_swtDrvNGovActv/1 -> BC/12  "testSig_DrvDem_swtDrvNGovActv"
  spec_PT_stTraRevGear/1 -> BC/13  "testSig_PT_stTraRevGear"
  spec_AccPed_trqLeadPull_mp/1 -> BC/14  "testSig_AccPed_trqLeadPull_mp"
  spec_AccPed_trqLeadOvrRun_mp/1 -> BC/15  "testSig_AccPed_trqLeadOvrRun_mp"
  spec_AccPed_trqLead/1 -> BC/16  "testSig_AccPed_trqLead"

== system TST_AccPed_DrvDemLead/simulationInput/testSignals_R002 ==
  BC : BusCreator  Inputs=16
  spec_APP_rUnFlt : FromWorkspace  VariableName=testSig_APP_rUnFlt  Interpolate=off  OutputAfterFinalValue=Holding final value
  spec_AccPed_rTrq : FromWorkspace  VariableName=testSig_AccPed_rTrq  Interpolate=off  OutputAfterFinalValue=Holding final value
  spec_AccPed_stBrkDes : FromWorkspace  VariableName=testSig_AccPed_stBrkDes  Interpolate=off  OutputAfterFinalValue=Holding final value
  spec_AccPed_stMS : FromWorkspace  VariableName=testSig_AccPed_stMS  Interpolate=off  OutputAfterFinalValue=Holding final value
  spec_AccPed_trqComp : FromWorkspace  VariableName=testSig_AccPed_trqComp  Interpolate=off  OutputAfterFinalValue=Holding final value
  spec_AccPed_trqDes : FromWorkspace  VariableName=testSig_AccPed_trqDes  Interpolate=off  OutputAfterFinalValue=Holding final value
  spec_AccPed_trqLead : FromWorkspace  VariableName=testSig_AccPed_trqLead  Interpolate=off  OutputAfterFinalValue=Holding final value
  spec_AccPed_trqLeadOvrRun_mp : FromWorkspace  VariableName=testSig_AccPed_trqLeadOvrRun_mp  Interpolate=off  OutputAfterFinalValue=Holding final value
  spec_AccPed_trqLeadPull_mp : FromWorkspace  VariableName=testSig_AccPed_trqLeadPull_mp  Interpolate=off  OutputAfterFinalValue=Holding final value
  spec_AccPed_trqLimMax : FromWorkspace  VariableName=testSig_AccPed_trqLimMax  Interpolate=off  OutputAfterFinalValue=Holding final value
  spec_CoME_trqDesComp : FromWorkspace  VariableName=testSig_CoME_trqDesComp  Interpolate=off  OutputAfterFinalValue=Holding final value
  spec_DrvDem_swtDrvNGovActv : FromWorkspace  VariableName=testSig_DrvDem_swtDrvNGovActv  Interpolate=off  OutputAfterFinalValue=Holding final value
  spec_Epm_nEng : FromWorkspace  VariableName=testSig_Epm_nEng  Interpolate=off  OutputAfterFinalValue=Holding final value
  spec_GlbDa_vX : FromWorkspace  VariableName=testSig_GlbDa_vX  Interpolate=off  OutputAfterFinalValue=Holding final value
  spec_PT_stTraRevGear : FromWorkspace  VariableName=testSig_PT_stTraRevGear  Interpolate=off  OutputAfterFinalValue=Holding final value
  spec_PT_trqWhlMinEng : FromWorkspace  VariableName=testSig_PT_trqWhlMinEng  Interpolate=off  OutputAfterFinalValue=Holding final value
  testSignals : Outport
  wires:
  BC/1 -> testSignals/1
  spec_PT_trqWhlMinEng/1 -> BC/1  "testSig_PT_trqWhlMinEng"
  spec_Epm_nEng/1 -> BC/2  "testSig_Epm_nEng"
  spec_AccPed_trqLimMax/1 -> BC/3  "testSig_AccPed_trqLimMax"
  spec_AccPed_rTrq/1 -> BC/4  "testSig_AccPed_rTrq"
  spec_AccPed_trqComp/1 -> BC/5  "testSig_AccPed_trqComp"
  spec_AccPed_stMS/1 -> BC/6  "testSig_AccPed_stMS"
  spec_APP_rUnFlt/1 -> BC/7  "testSig_APP_rUnFlt"
  spec_AccPed_trqDes/1 -> BC/8  "testSig_AccPed_trqDes"
  spec_CoME_trqDesComp/1 -> BC/9  "testSig_CoME_trqDesComp"
  spec_GlbDa_vX/1 -> BC/10  "testSig_GlbDa_vX"
  spec_AccPed_stBrkDes/1 -> BC/11  "testSig_AccPed_stBrkDes"
  spec_DrvDem_swtDrvNGovActv/1 -> BC/12  "testSig_DrvDem_swtDrvNGovActv"
  spec_PT_stTraRevGear/1 -> BC/13  "testSig_PT_stTraRevGear"
  spec_AccPed_trqLeadPull_mp/1 -> BC/14  "testSig_AccPed_trqLeadPull_mp"
  spec_AccPed_trqLeadOvrRun_mp/1 -> BC/15  "testSig_AccPed_trqLeadOvrRun_mp"
  spec_AccPed_trqLead/1 -> BC/16  "testSig_AccPed_trqLead"

== system TST_AccPed_DrvDemLead/simulationInput/testSignals_R003 ==
  BC : BusCreator  Inputs=16
  spec_APP_rUnFlt : FromWorkspace  VariableName=testSig_APP_rUnFlt  Interpolate=off  OutputAfterFinalValue=Holding final value
  spec_AccPed_rTrq : FromWorkspace  VariableName=testSig_AccPed_rTrq  Interpolate=off  OutputAfterFinalValue=Holding final value
  spec_AccPed_stBrkDes : FromWorkspace  VariableName=testSig_AccPed_stBrkDes  Interpolate=off  OutputAfterFinalValue=Holding final value
  spec_AccPed_stMS : FromWorkspace  VariableName=testSig_AccPed_stMS  Interpolate=off  OutputAfterFinalValue=Holding final value
  spec_AccPed_trqComp : FromWorkspace  VariableName=testSig_AccPed_trqComp  Interpolate=off  OutputAfterFinalValue=Holding final value
  spec_AccPed_trqDes : FromWorkspace  VariableName=testSig_AccPed_trqDes  Interpolate=off  OutputAfterFinalValue=Holding final value
  spec_AccPed_trqLead : FromWorkspace  VariableName=testSig_AccPed_trqLead  Interpolate=off  OutputAfterFinalValue=Holding final value
  spec_AccPed_trqLeadOvrRun_mp : FromWorkspace  VariableName=testSig_AccPed_trqLeadOvrRun_mp  Interpolate=off  OutputAfterFinalValue=Holding final value
  spec_AccPed_trqLeadPull_mp : FromWorkspace  VariableName=testSig_AccPed_trqLeadPull_mp  Interpolate=off  OutputAfterFinalValue=Holding final value
  spec_AccPed_trqLimMax : FromWorkspace  VariableName=testSig_AccPed_trqLimMax  Interpolate=off  OutputAfterFinalValue=Holding final value
  spec_CoME_trqDesComp : FromWorkspace  VariableName=testSig_CoME_trqDesComp  Interpolate=off  OutputAfterFinalValue=Holding final value
  spec_DrvDem_swtDrvNGovActv : FromWorkspace  VariableName=testSig_DrvDem_swtDrvNGovActv  Interpolate=off  OutputAfterFinalValue=Holding final value
  spec_Epm_nEng : FromWorkspace  VariableName=testSig_Epm_nEng  Interpolate=off  OutputAfterFinalValue=Holding final value
  spec_GlbDa_vX : FromWorkspace  VariableName=testSig_GlbDa_vX  Interpolate=off  OutputAfterFinalValue=Holding final value
  spec_PT_stTraRevGear : FromWorkspace  VariableName=testSig_PT_stTraRevGear  Interpolate=off  OutputAfterFinalValue=Holding final value
  spec_PT_trqWhlMinEng : FromWorkspace  VariableName=testSig_PT_trqWhlMinEng  Interpolate=off  OutputAfterFinalValue=Holding final value
  testSignals : Outport
  wires:
  BC/1 -> testSignals/1
  spec_PT_trqWhlMinEng/1 -> BC/1  "testSig_PT_trqWhlMinEng"
  spec_Epm_nEng/1 -> BC/2  "testSig_Epm_nEng"
  spec_AccPed_trqLimMax/1 -> BC/3  "testSig_AccPed_trqLimMax"
  spec_AccPed_rTrq/1 -> BC/4  "testSig_AccPed_rTrq"
  spec_AccPed_trqComp/1 -> BC/5  "testSig_AccPed_trqComp"
  spec_AccPed_stMS/1 -> BC/6  "testSig_AccPed_stMS"
  spec_APP_rUnFlt/1 -> BC/7  "testSig_APP_rUnFlt"
  spec_AccPed_trqDes/1 -> BC/8  "testSig_AccPed_trqDes"
  spec_CoME_trqDesComp/1 -> BC/9  "testSig_CoME_trqDesComp"
  spec_GlbDa_vX/1 -> BC/10  "testSig_GlbDa_vX"
  spec_AccPed_stBrkDes/1 -> BC/11  "testSig_AccPed_stBrkDes"
  spec_DrvDem_swtDrvNGovActv/1 -> BC/12  "testSig_DrvDem_swtDrvNGovActv"
  spec_PT_stTraRevGear/1 -> BC/13  "testSig_PT_stTraRevGear"
  spec_AccPed_trqLeadPull_mp/1 -> BC/14  "testSig_AccPed_trqLeadPull_mp"
  spec_AccPed_trqLeadOvrRun_mp/1 -> BC/15  "testSig_AccPed_trqLeadOvrRun_mp"
  spec_AccPed_trqLead/1 -> BC/16  "testSig_AccPed_trqLead"

== system TST_AccPed_DrvDemLead/simulationInput/testSignals_R004 ==
  BC : BusCreator  Inputs=16
  spec_APP_rUnFlt : FromWorkspace  VariableName=testSig_APP_rUnFlt  Interpolate=off  OutputAfterFinalValue=Holding final value
  spec_AccPed_rTrq : FromWorkspace  VariableName=testSig_AccPed_rTrq  Interpolate=off  OutputAfterFinalValue=Holding final value
  spec_AccPed_stBrkDes : FromWorkspace  VariableName=testSig_AccPed_stBrkDes  Interpolate=off  OutputAfterFinalValue=Holding final value
  spec_AccPed_stMS : FromWorkspace  VariableName=testSig_AccPed_stMS  Interpolate=off  OutputAfterFinalValue=Holding final value
  spec_AccPed_trqComp : FromWorkspace  VariableName=testSig_AccPed_trqComp  Interpolate=off  OutputAfterFinalValue=Holding final value
  spec_AccPed_trqDes : FromWorkspace  VariableName=testSig_AccPed_trqDes  Interpolate=off  OutputAfterFinalValue=Holding final value
  spec_AccPed_trqLead : FromWorkspace  VariableName=testSig_AccPed_trqLead  Interpolate=off  OutputAfterFinalValue=Holding final value
  spec_AccPed_trqLeadOvrRun_mp : FromWorkspace  VariableName=testSig_AccPed_trqLeadOvrRun_mp  Interpolate=off  OutputAfterFinalValue=Holding final value
  spec_AccPed_trqLeadPull_mp : FromWorkspace  VariableName=testSig_AccPed_trqLeadPull_mp  Interpolate=off  OutputAfterFinalValue=Holding final value
  spec_AccPed_trqLimMax : FromWorkspace  VariableName=testSig_AccPed_trqLimMax  Interpolate=off  OutputAfterFinalValue=Holding final value
  spec_CoME_trqDesComp : FromWorkspace  VariableName=testSig_CoME_trqDesComp  Interpolate=off  OutputAfterFinalValue=Holding final value
  spec_DrvDem_swtDrvNGovActv : FromWorkspace  VariableName=testSig_DrvDem_swtDrvNGovActv  Interpolate=off  OutputAfterFinalValue=Holding final value
  spec_Epm_nEng : FromWorkspace  VariableName=testSig_Epm_nEng  Interpolate=off  OutputAfterFinalValue=Holding final value
  spec_GlbDa_vX : FromWorkspace  VariableName=testSig_GlbDa_vX  Interpolate=off  OutputAfterFinalValue=Holding final value
  spec_PT_stTraRevGear : FromWorkspace  VariableName=testSig_PT_stTraRevGear  Interpolate=off  OutputAfterFinalValue=Holding final value
  spec_PT_trqWhlMinEng : FromWorkspace  VariableName=testSig_PT_trqWhlMinEng  Interpolate=off  OutputAfterFinalValue=Holding final value
  testSignals : Outport
  wires:
  BC/1 -> testSignals/1
  spec_PT_trqWhlMinEng/1 -> BC/1  "testSig_PT_trqWhlMinEng"
  spec_Epm_nEng/1 -> BC/2  "testSig_Epm_nEng"
  spec_AccPed_trqLimMax/1 -> BC/3  "testSig_AccPed_trqLimMax"
  spec_AccPed_rTrq/1 -> BC/4  "testSig_AccPed_rTrq"
  spec_AccPed_trqComp/1 -> BC/5  "testSig_AccPed_trqComp"
  spec_AccPed_stMS/1 -> BC/6  "testSig_AccPed_stMS"
  spec_APP_rUnFlt/1 -> BC/7  "testSig_APP_rUnFlt"
  spec_AccPed_trqDes/1 -> BC/8  "testSig_AccPed_trqDes"
  spec_CoME_trqDesComp/1 -> BC/9  "testSig_CoME_trqDesComp"
  spec_GlbDa_vX/1 -> BC/10  "testSig_GlbDa_vX"
  spec_AccPed_stBrkDes/1 -> BC/11  "testSig_AccPed_stBrkDes"
  spec_DrvDem_swtDrvNGovActv/1 -> BC/12  "testSig_DrvDem_swtDrvNGovActv"
  spec_PT_stTraRevGear/1 -> BC/13  "testSig_PT_stTraRevGear"
  spec_AccPed_trqLeadPull_mp/1 -> BC/14  "testSig_AccPed_trqLeadPull_mp"
  spec_AccPed_trqLeadOvrRun_mp/1 -> BC/15  "testSig_AccPed_trqLeadOvrRun_mp"
  spec_AccPed_trqLead/1 -> BC/16  "testSig_AccPed_trqLead"

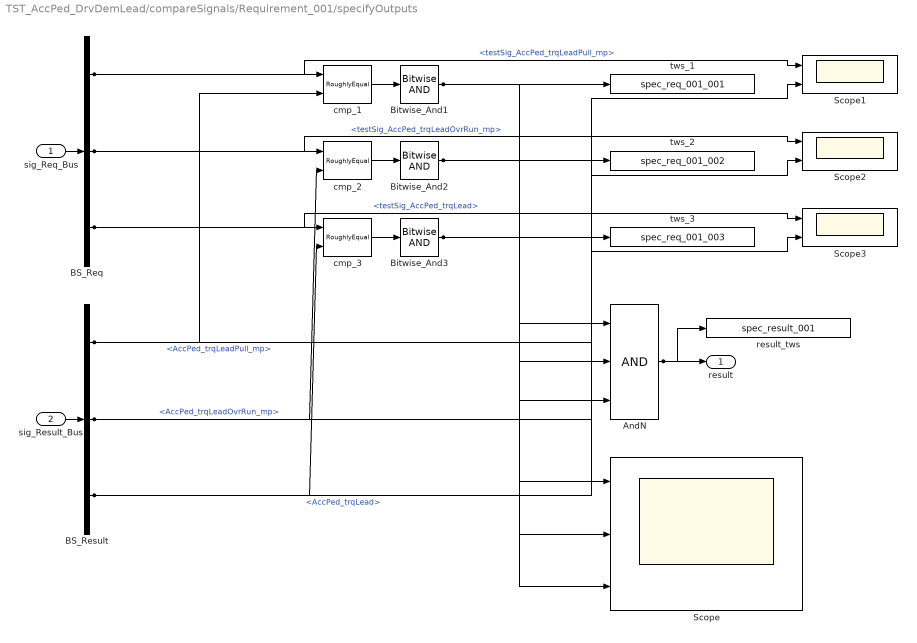
== system TST_AccPed_DrvDemLead/compareSignals/Requirement_001/specifyOutputs ==
  sig_Req_Bus : Inport
  sig_Result_Bus : Inport  Port=2
  AndN : Logic  Inputs=3
  BS_Req : BusSelector  OutputSignals=testSig_AccPed_trqLeadPull_mp,testSig_AccPed_trqLeadOvrRun_mp,testSig_AccPed_trqLead
  BS_Result : BusSelector  OutputSignals=AccPed_trqLeadPull_mp,AccPed_trqLeadOvrRun_mp,AccPed_trqLead
  Bitwise_And1 : simulink/Logic and Bit Operations/Bitwise Operator  logicop=AND  UseBitMask=off  BitMask=bin2dec('11011001')  BitMaskRealWorld=Stored Integer
  Bitwise_And2 : simulink/Logic and Bit Operations/Bitwise Operator  logicop=AND  UseBitMask=off  BitMask=bin2dec('11011001')  BitMaskRealWorld=Stored Integer
  Bitwise_And3 : simulink/Logic and Bit Operations/Bitwise Operator  logicop=AND  UseBitMask=off  BitMask=bin2dec('11011001')  BitMaskRealWorld=Stored Integer
  Scope : Scope  NumInputPorts=3
  Scope1 : Scope  NumInputPorts=2
  Scope2 : Scope  NumInputPorts=2
  Scope3 : Scope  NumInputPorts=2
  cmp_1 : UnitTest_Lib/RoughlyEqual  slope=0.1
  cmp_2 : UnitTest_Lib/RoughlyEqual  slope=0.1
  cmp_3 : UnitTest_Lib/RoughlyEqual  slope=0.1
  result_tws : ToWorkspace  VariableName=spec_result_001
  tws_1 : ToWorkspace  VariableName=spec_req_001_001
  tws_2 : ToWorkspace  VariableName=spec_req_001_002
  tws_3 : ToWorkspace  VariableName=spec_req_001_003
  result : Outport
  wires:
  sig_Req_Bus/1 -> BS_Req/1
  sig_Result_Bus/1 -> BS_Result/1
  AndN/1 -> result/1, result_tws/1
  BS_Req/1 -> cmp_1/1, Scope1/1  "<testSig_AccPed_trqLeadPull_mp>"
  BS_Result/1 -> cmp_1/2, Scope1/2  "<AccPed_trqLeadPull_mp>"
  cmp_1/1 -> Bitwise_And1/1
  Bitwise_And1/1 -> tws_1/1, AndN/1, Scope/1
  BS_Req/2 -> cmp_2/1, Scope2/1  "<testSig_AccPed_trqLeadOvrRun_mp>"
  BS_Result/2 -> cmp_2/2, Scope2/2  "<AccPed_trqLeadOvrRun_mp>"
  cmp_2/1 -> Bitwise_And2/1
  Bitwise_And2/1 -> tws_2/1, AndN/2, Scope/2
  BS_Req/3 -> cmp_3/1, Scope3/1  "<testSig_AccPed_trqLead>"
  BS_Result/3 -> cmp_3/2, Scope3/2  "<AccPed_trqLead>"
  cmp_3/1 -> Bitwise_And3/1
  Bitwise_And3/1 -> tws_3/1, AndN/3, Scope/3

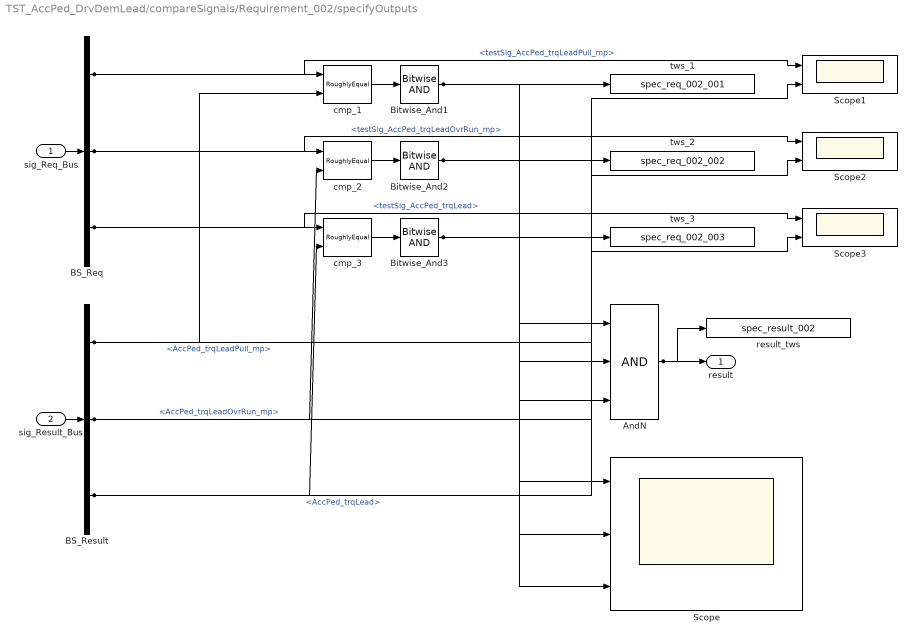
== system TST_AccPed_DrvDemLead/compareSignals/Requirement_002/specifyOutputs ==
  sig_Req_Bus : Inport
  sig_Result_Bus : Inport  Port=2
  AndN : Logic  Inputs=3
  BS_Req : BusSelector  OutputSignals=testSig_AccPed_trqLeadPull_mp,testSig_AccPed_trqLeadOvrRun_mp,testSig_AccPed_trqLead
  BS_Result : BusSelector  OutputSignals=AccPed_trqLeadPull_mp,AccPed_trqLeadOvrRun_mp,AccPed_trqLead
  Bitwise_And1 : simulink/Logic and Bit Operations/Bitwise Operator  logicop=AND  UseBitMask=off  BitMask=bin2dec('11011001')  BitMaskRealWorld=Stored Integer
  Bitwise_And2 : simulink/Logic and Bit Operations/Bitwise Operator  logicop=AND  UseBitMask=off  BitMask=bin2dec('11011001')  BitMaskRealWorld=Stored Integer
  Bitwise_And3 : simulink/Logic and Bit Operations/Bitwise Operator  logicop=AND  UseBitMask=off  BitMask=bin2dec('11011001')  BitMaskRealWorld=Stored Integer
  Scope : Scope  NumInputPorts=3
  Scope1 : Scope  NumInputPorts=2
  Scope2 : Scope  NumInputPorts=2
  Scope3 : Scope  NumInputPorts=2
  cmp_1 : UnitTest_Lib/RoughlyEqual  slope=0.1
  cmp_2 : UnitTest_Lib/RoughlyEqual  slope=0.1
  cmp_3 : UnitTest_Lib/RoughlyEqual  slope=0.1
  result_tws : ToWorkspace  VariableName=spec_result_002
  tws_1 : ToWorkspace  VariableName=spec_req_002_001
  tws_2 : ToWorkspace  VariableName=spec_req_002_002
  tws_3 : ToWorkspace  VariableName=spec_req_002_003
  result : Outport
  wires:
  sig_Req_Bus/1 -> BS_Req/1
  sig_Result_Bus/1 -> BS_Result/1
  AndN/1 -> result/1, result_tws/1
  BS_Req/1 -> cmp_1/1, Scope1/1  "<testSig_AccPed_trqLeadPull_mp>"
  BS_Result/1 -> cmp_1/2, Scope1/2  "<AccPed_trqLeadPull_mp>"
  cmp_1/1 -> Bitwise_And1/1
  Bitwise_And1/1 -> tws_1/1, AndN/1, Scope/1
  BS_Req/2 -> cmp_2/1, Scope2/1  "<testSig_AccPed_trqLeadOvrRun_mp>"
  BS_Result/2 -> cmp_2/2, Scope2/2  "<AccPed_trqLeadOvrRun_mp>"
  cmp_2/1 -> Bitwise_And2/1
  Bitwise_And2/1 -> tws_2/1, AndN/2, Scope/2
  BS_Req/3 -> cmp_3/1, Scope3/1  "<testSig_AccPed_trqLead>"
  BS_Result/3 -> cmp_3/2, Scope3/2  "<AccPed_trqLead>"
  cmp_3/1 -> Bitwise_And3/1
  Bitwise_And3/1 -> tws_3/1, AndN/3, Scope/3

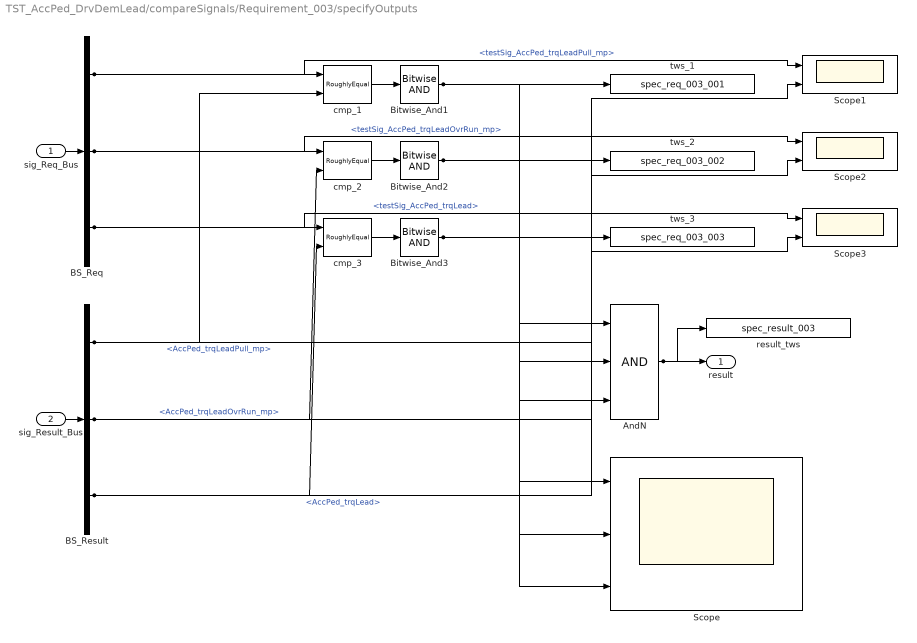
== system TST_AccPed_DrvDemLead/compareSignals/Requirement_003/specifyOutputs ==
  sig_Req_Bus : Inport
  sig_Result_Bus : Inport  Port=2
  AndN : Logic  Inputs=3
  BS_Req : BusSelector  OutputSignals=testSig_AccPed_trqLeadPull_mp,testSig_AccPed_trqLeadOvrRun_mp,testSig_AccPed_trqLead
  BS_Result : BusSelector  OutputSignals=AccPed_trqLeadPull_mp,AccPed_trqLeadOvrRun_mp,AccPed_trqLead
  Bitwise_And1 : simulink/Logic and Bit Operations/Bitwise Operator  logicop=AND  UseBitMask=off  BitMask=bin2dec('11011001')  BitMaskRealWorld=Stored Integer
  Bitwise_And2 : simulink/Logic and Bit Operations/Bitwise Operator  logicop=AND  UseBitMask=off  BitMask=bin2dec('11011001')  BitMaskRealWorld=Stored Integer
  Bitwise_And3 : simulink/Logic and Bit Operations/Bitwise Operator  logicop=AND  UseBitMask=off  BitMask=bin2dec('11011001')  BitMaskRealWorld=Stored Integer
  Scope : Scope  NumInputPorts=3
  Scope1 : Scope  NumInputPorts=2
  Scope2 : Scope  NumInputPorts=2
  Scope3 : Scope  NumInputPorts=2
  cmp_1 : UnitTest_Lib/RoughlyEqual  slope=0.1
  cmp_2 : UnitTest_Lib/RoughlyEqual  slope=0.1
  cmp_3 : UnitTest_Lib/RoughlyEqual  slope=0.1
  result_tws : ToWorkspace  VariableName=spec_result_003
  tws_1 : ToWorkspace  VariableName=spec_req_003_001
  tws_2 : ToWorkspace  VariableName=spec_req_003_002
  tws_3 : ToWorkspace  VariableName=spec_req_003_003
  result : Outport
  wires:
  sig_Req_Bus/1 -> BS_Req/1
  sig_Result_Bus/1 -> BS_Result/1
  AndN/1 -> result/1, result_tws/1
  BS_Req/1 -> cmp_1/1, Scope1/1  "<testSig_AccPed_trqLeadPull_mp>"
  BS_Result/1 -> cmp_1/2, Scope1/2  "<AccPed_trqLeadPull_mp>"
  cmp_1/1 -> Bitwise_And1/1
  Bitwise_And1/1 -> tws_1/1, AndN/1, Scope/1
  BS_Req/2 -> cmp_2/1, Scope2/1  "<testSig_AccPed_trqLeadOvrRun_mp>"
  BS_Result/2 -> cmp_2/2, Scope2/2  "<AccPed_trqLeadOvrRun_mp>"
  cmp_2/1 -> Bitwise_And2/1
  Bitwise_And2/1 -> tws_2/1, AndN/2, Scope/2
  BS_Req/3 -> cmp_3/1, Scope3/1  "<testSig_AccPed_trqLead>"
  BS_Result/3 -> cmp_3/2, Scope3/2  "<AccPed_trqLead>"
  cmp_3/1 -> Bitwise_And3/1
  Bitwise_And3/1 -> tws_3/1, AndN/3, Scope/3

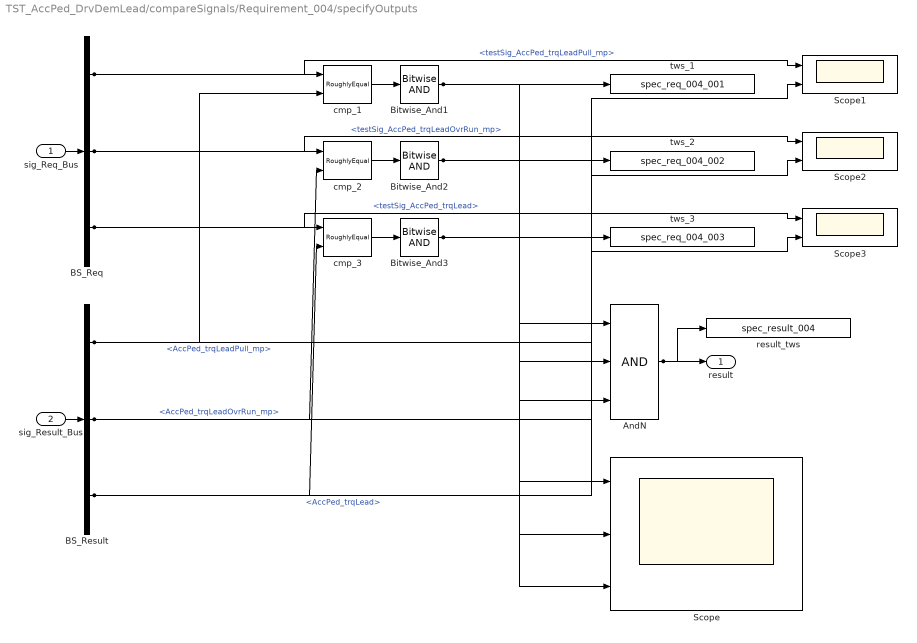
== system TST_AccPed_DrvDemLead/compareSignals/Requirement_004/specifyOutputs ==
  sig_Req_Bus : Inport
  sig_Result_Bus : Inport  Port=2
  AndN : Logic  Inputs=3
  BS_Req : BusSelector  OutputSignals=testSig_AccPed_trqLeadPull_mp,testSig_AccPed_trqLeadOvrRun_mp,testSig_AccPed_trqLead
  BS_Result : BusSelector  OutputSignals=AccPed_trqLeadPull_mp,AccPed_trqLeadOvrRun_mp,AccPed_trqLead
  Bitwise_And1 : simulink/Logic and Bit Operations/Bitwise Operator  logicop=AND  UseBitMask=off  BitMask=bin2dec('11011001')  BitMaskRealWorld=Stored Integer
  Bitwise_And2 : simulink/Logic and Bit Operations/Bitwise Operator  logicop=AND  UseBitMask=off  BitMask=bin2dec('11011001')  BitMaskRealWorld=Stored Integer
  Bitwise_And3 : simulink/Logic and Bit Operations/Bitwise Operator  logicop=AND  UseBitMask=off  BitMask=bin2dec('11011001')  BitMaskRealWorld=Stored Integer
  Scope : Scope  NumInputPorts=3
  Scope1 : Scope  NumInputPorts=2
  Scope2 : Scope  NumInputPorts=2
  Scope3 : Scope  NumInputPorts=2
  cmp_1 : UnitTest_Lib/RoughlyEqual  slope=0.1
  cmp_2 : UnitTest_Lib/RoughlyEqual  slope=0.1
  cmp_3 : UnitTest_Lib/RoughlyEqual  slope=0.1
  result_tws : ToWorkspace  VariableName=spec_result_004
  tws_1 : ToWorkspace  VariableName=spec_req_004_001
  tws_2 : ToWorkspace  VariableName=spec_req_004_002
  tws_3 : ToWorkspace  VariableName=spec_req_004_003
  result : Outport
  wires:
  sig_Req_Bus/1 -> BS_Req/1
  sig_Result_Bus/1 -> BS_Result/1
  AndN/1 -> result/1, result_tws/1
  BS_Req/1 -> cmp_1/1, Scope1/1  "<testSig_AccPed_trqLeadPull_mp>"
  BS_Result/1 -> cmp_1/2, Scope1/2  "<AccPed_trqLeadPull_mp>"
  cmp_1/1 -> Bitwise_And1/1
  Bitwise_And1/1 -> tws_1/1, AndN/1, Scope/1
  BS_Req/2 -> cmp_2/1, Scope2/1  "<testSig_AccPed_trqLeadOvrRun_mp>"
  BS_Result/2 -> cmp_2/2, Scope2/2  "<AccPed_trqLeadOvrRun_mp>"
  cmp_2/1 -> Bitwise_And2/1
  Bitwise_And2/1 -> tws_2/1, AndN/2, Scope/2
  BS_Req/3 -> cmp_3/1, Scope3/1  "<testSig_AccPed_trqLead>"
  BS_Result/3 -> cmp_3/2, Scope3/2  "<AccPed_trqLead>"
  cmp_3/1 -> Bitwise_And3/1
  Bitwise_And3/1 -> tws_3/1, AndN/3, Scope/3
